simulink model "problem_6"  (R2023b)
settings: Solver=VariableStepAuto  StartTime=0.0  StopTime=10.0  RelTol=1e-3
settings Model: Creator=Sasha  LastModifiedBy=Sasha

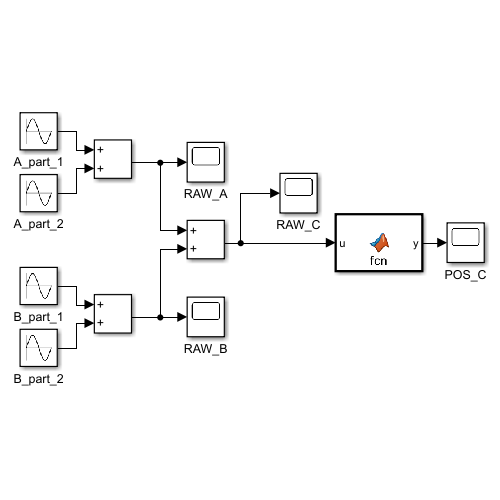
[thumbnail: Simulink's stored preview of the top-level diagram]
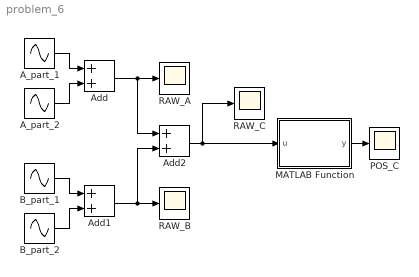
== system problem_6 ==
  A_part_1 : Sin  Amplitude=5  Frequency=279145/20000  SampleTime=0
  A_part_2 : Sin  SampleTime=0
  Add : Sum
  Add1 : Sum
  Add2 : Sum
  B_part_1 : Sin  Amplitude=10  Frequency=279145/30000  Phase=279145*pi/60000  SampleTime=0
  B_part_2 : Sin  Phase=-pi/2  SampleTime=0
  MATLAB Function : MATLAB Function  TreatAsAtomicUnit=on
  POS_C : Scope
  RAW_A : Scope
  RAW_B : Scope
  RAW_C : Scope
  wires:
  A_part_1/1 -> Add/1
  A_part_2/1 -> Add/2
  B_part_1/1 -> Add1/1
  B_part_2/1 -> Add1/2
  Add/1 -> RAW_A/1, Add2/1
  Add1/1 -> RAW_B/1, Add2/2
  MATLAB Function/1(y) -> POS_C/1
  Add2/1 -> RAW_C/1, MATLAB Function/1(u)

== matlab function problem_6/MATLAB Function ==
  data: u input; y output
function y = fcn(u)
    y = max(0, u);
end
